simulink model "euler_dynamics"  (R2024b)
settings: Solver=FixedStepAuto  StartTime=0.0  StopTime=1500  FixedStep=0.1  RelTol=1e-6  AbsTol=1e-6
values from neighbouring files (symbols this model uses):
  com_0 = [0,0,0]    [Specefications.m]
  com_1 = [60,60,60]*deg    [Specefications.m]
  com_2 = [-60,-60,-60]*deg    [Specefications.m]
  com_3 = [0,0,0]*deg    [Specefications.m]
  deg = pi/180    (= 0.0174532925199)    [Specefications.m]
  initial_euler_angles = [30,30,30].*deg    [Specefications.m]
  J = diag([J11,J22,J33])    [Specefications.m]
  K_e = lqr(Linearized_model_e,Q,R)    [Linear_controller_design.m]
  n = (mu_Earth/r^3).^0.5    [Specefications.m]
  t_d = [1e-4,1e-4,1e-4]    [Specefications.m]
  w = [0,0,0].*deg    [Specefications.m]
libraries: matrix_library x2, sharedtransform x2
settings Model: Creator=diogo  LastModifiedBy=diogo

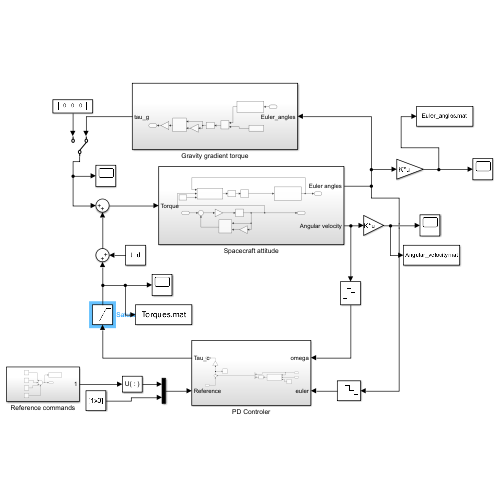
[thumbnail: Simulink's stored preview of the top-level diagram]
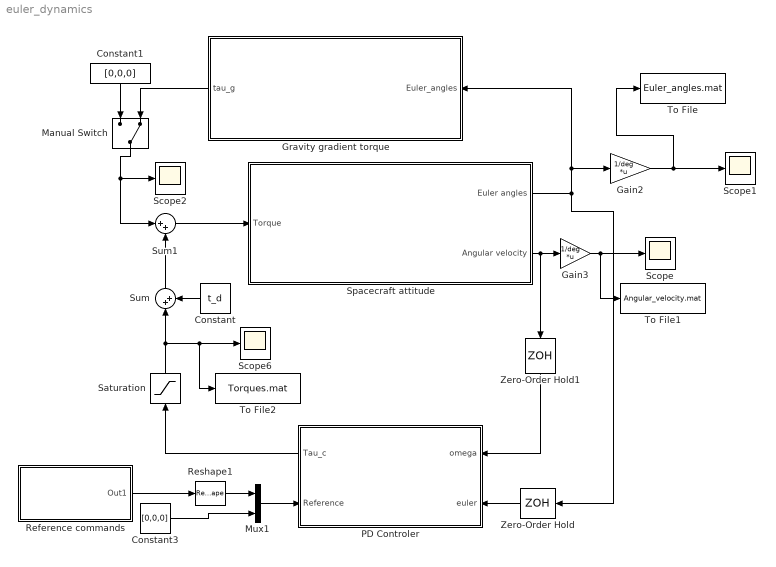
== system euler_dynamics ==
  Constant : Constant  Value=t_d
  Constant1 : Constant  Value=[0,0,0]
  Constant3 : Constant  Value=[0,0,0]
  Gain2 : Gain  Gain=1/deg  Multiplication=Matrix(K*u)
  Gain3 : Gain  Gain=1/deg  Multiplication=Matrix(K*u)
  Gravity gradient torque : Subsystem
  Manual Switch : ManualSwitch  CurrentSetting=0
  Mux1 : Mux  Inputs=2
  PD Controler : Subsystem
      settings: PortSchema="{\"entries\":[{\"content\":{\"sides\":[{\"content\":{\"connectorIds\":[\"Out1\",\"In1\"]},\"type\":\"ConnectorPlacement.EquallySpacedRectSide\",\"uuid\":\"f595316a-67fa-4e45-afef-328468ac5eb6\"},{\"content\":{\"connectorIds\":[\"In2\",\"In3\"],\"side\":\"RIGHT\"},\"type\":\"ConnectorPlacement.EquallySpacedRectSide\",\"uuid\":\"1d08d35b-debb-44a1-b4ca-ee5ff70ce730\"},{\"content\":{\"side\":\"TOP\"},\"type\":\"ConnectorPlacement.EquallySpacedRectSide\",\"uuid\":\"f0dda074-91f8-4f2d-97e8-f0eac84287d6\"}]},\"type\":\"ConnectorPlacement.EquallySpacedConnector\",\"uuid\":\"e9b94e59-1199-495c-ac6d-8aec278c5c81\"}],\"packageUris\":[\"http://schema.mathworks.com/mf0/Connector/R2020b\"],\"version\":\"1.0\"}"
  Reference commands : Subsystem
  Reshape1 : Reshape
  Saturation : Saturate  UpperLimit=1  LowerLimit=-1
  Scope{,1..2,6} (4 alike) : Scope
  Spacecraft attitude : Subsystem
  Sum : Sum  Inputs=|++
  Sum1 : Sum  Inputs=|++
  To File : ToFile  Filename=Euler_angles.mat  MatrixName=values  SaveFormat=Timeseries
  To File1 : ToFile  Filename=Angular_velocity.mat  MatrixName=values  SaveFormat=Timeseries
  To File2 : ToFile  Filename=Torques.mat  MatrixName=values  SaveFormat=Timeseries
  Zero-Order Hold : ZeroOrderHold  SampleTime=0.1
  Zero-Order Hold1 : ZeroOrderHold  SampleTime=0.1
  wires:
  Gain3/1 -> To File1/1, Scope/1
  Spacecraft attitude/2(Angular velocity) -> Zero-Order Hold1/1, Gain3/1
  Constant/1 -> Sum/2
  Sum/1 -> Sum1/2
  Sum1/1 -> Spacecraft attitude/1(Torque)
  Gain2/1 -> To File/1, Scope1/1
  Constant1/1 -> Manual Switch/1
  Gravity gradient torque/1(tau_g) -> Manual Switch/2
  Manual Switch/1 -> Sum1/1, Scope2/1
  Spacecraft attitude/1(Euler angles) -> Gain2/1, Gravity gradient torque/1(Euler_angles), Zero-Order Hold/1
  Reference commands/1(Out1) -> Reshape1/1
  Reshape1/1 -> Mux1/1
  Constant3/1 -> Mux1/2
  PD Controler/1(Tau_c) -> Saturation/1
  Zero-Order Hold1/1 -> PD Controler/2(omega)
  Zero-Order Hold/1 -> PD Controler/3(euler)
  Mux1/1 -> PD Controler/1(Reference)
  Saturation/1 -> Sum/1, To File2/1, Scope6/1

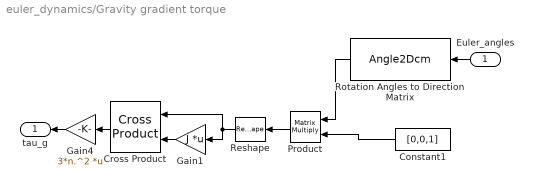
== system euler_dynamics/Gravity gradient torque ==
  Euler_angles : Inport
  Constant1 : Constant  Value=[0,0,1]
  Cross Product : matrix_library/Cross Product
  Gain1 : Gain  Gain=J  Multiplication=Matrix(K*u)
  Gain4 : Gain  Gain=3*n.^2  Multiplication=Matrix(K*u)
  Product : Product  Multiplication=Matrix(*)
  Reshape : Reshape
  Rotation Angles to Direction  Matrix : Angle2Dcm
      settings: AttributesFormatString=Rotation Order: %<rotationOrder>
  tau_g : Outport
  wires:
  Constant1/1 -> Product/2
  Gain1/1 -> Cross Product/2
  Gain4/1 -> tau_g/1
  Cross Product/1 -> Gain4/1
  Euler_angles/1 -> Rotation Angles to Direction  Matrix/1
  Product/1 -> Reshape/1
  Reshape/1 -> Gain1/1, Cross Product/1
  Rotation Angles to Direction  Matrix/1 -> Product/1

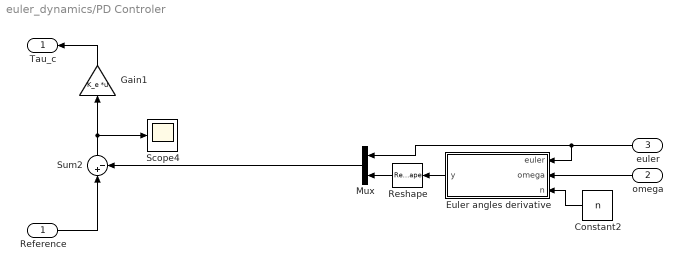
== system euler_dynamics/PD Controler ==
  Reference : Inport
  omega : Inport  Port=2
  euler : Inport  Port=3
  Constant2 : Constant  Value=n
  Euler angles derivative : MATLAB Function  TreatAsAtomicUnit=on
  Gain1 : Gain  Gain=K_e  Multiplication=Matrix(K*u)
  Mux : Mux  Inputs=2
  Reshape : Reshape
  Scope4 : Scope
  Sum2 : Sum  Inputs=|+-
  Tau_c : Outport
  wires:
  Sum2/1 -> Scope4/1, Gain1/1
  Constant2/1 -> Euler angles derivative/3(n)
  Mux/1 -> Sum2/2
  euler/1 -> Mux/1, Euler angles derivative/1(euler)
  Reshape/1 -> Mux/2
  Euler angles derivative/1(y) -> Reshape/1
  Gain1/1 -> Tau_c/1
  omega/1 -> Euler angles derivative/2(omega)
  Reference/1 -> Sum2/1

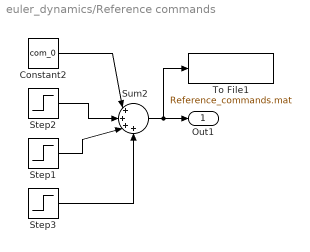
== system euler_dynamics/Reference commands ==
  Constant2 : Constant  Value=com_0
  Step1 : Step  Time=500.1  After=com_2 - com_1  SampleTime=0  VectorParams1D=off
  Step2 : Step  Time=100  After=com_1 - com_0  SampleTime=0  VectorParams1D=off
  Step3 : Step  Time=900.1  After=com_3 - com_2  SampleTime=0  VectorParams1D=off
  Sum2 : Sum  Inputs=|++++
  To File1 : ToFile  Filename=Reference_commands.mat  MatrixName=values  SaveFormat=Timeseries
  Out1 : Outport
  wires:
  Step3/1 -> Sum2/4
  Step1/1 -> Sum2/3
  Step2/1 -> Sum2/2
  Constant2/1 -> Sum2/1
  Sum2/1 -> To File1/1, Out1/1

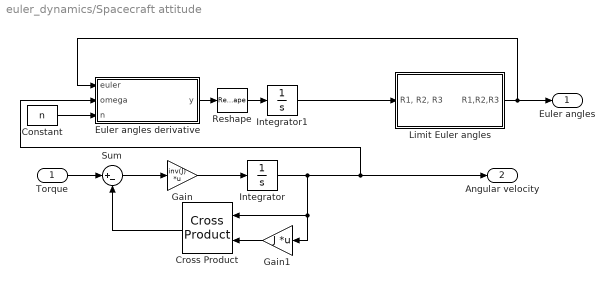
== system euler_dynamics/Spacecraft attitude ==
  Torque : Inport
  Constant : Constant  Value=n
  Cross Product : matrix_library/Cross Product
  Euler angles derivative : MATLAB Function  TreatAsAtomicUnit=on
  Gain : Gain  Gain=inv(J)  Multiplication=Matrix(K*u)
  Gain1 : Gain  Gain=J  Multiplication=Matrix(K*u)
  Integrator : Integrator  InitialCondition=w
  Integrator1 : Integrator  InitialCondition=initial_euler_angles
  Limit Euler angles : Subsystem
  Reshape : Reshape
  Sum : Sum  Inputs=|+-
  Euler angles : Outport
  Angular velocity : Outport  Port=2
  wires:
  Gain1/1 -> Cross Product/2
  Integrator/1 -> Cross Product/1, Gain1/1, Euler angles derivative/2(omega), Angular velocity/1
  Sum/1 -> Gain/1
  Cross Product/1 -> Sum/2
  Gain/1 -> Integrator/1
  Torque/1 -> Sum/1
  Euler angles derivative/1(y) -> Reshape/1
  Integrator1/1 -> Limit Euler angles/1("R1, R2, R3")
  Constant/1 -> Euler angles derivative/3(n)
  Limit Euler angles/1(R1,R2,R3) -> Euler angles derivative/1(euler), Euler angles/1
  Reshape/1 -> Integrator1/1

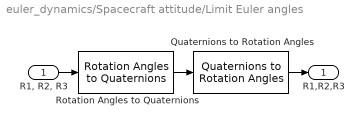
== system euler_dynamics/Spacecraft attitude/Limit Euler angles ==
  "R1, R2, R3" : Inport
  Quaternions to Rotation Angles : sharedtransform/Quaternions to Rotation Angles  rotationOrder=ZYX  aMode=aMode
  Rotation Angles to Quaternions : sharedtransform/Rotation Angles to Quaternions  rotationOrder=ZYX  aMode=aMode
  R1,R2,R3 : Outport
  wires:
  Quaternions to Rotation Angles/1 -> R1,R2,R3/1
  Rotation Angles to Quaternions/1 -> Quaternions to Rotation Angles/1
  "R1, R2, R3"/1 -> Rotation Angles to Quaternions/1

== matlab function euler_dynamics/Spacecraft attitude/Euler angles derivative ==
  data: euler input; y output; omega input; n input
function y = fcn(euler,omega,n)
theta = euler(2);
phi = euler(3);
psi = euler(1);
mat = (1/cos(theta))*[cos(theta),sin(phi)*sin(theta),cos(phi)*sin(theta);
0, cos(phi)*cos(theta),-sin(phi)*cos(theta);
0, sin(phi), cos(phi)
];
z = mat*omega + n/cos(theta)*[sin(psi); cos(theta)*cos(psi); sin(theta)*sin(psi)];
y = [z(3),z(2),z(1)];

== matlab function euler_dynamics/PD Controler/Euler angles derivative ==
  data: euler input; y output; omega input; n input
function y = fcn(euler,omega,n)
theta = euler(2);
phi = euler(3);
psi = euler(1);
mat = (1/cos(theta))*[cos(theta),sin(phi)*sin(theta),cos(phi)*sin(theta);
0, cos(phi)*cos(theta),-sin(phi)*cos(theta);
0, sin(phi), cos(phi)
];
z = mat*omega + n/cos(theta)*[sin(psi); cos(theta)*cos(psi); sin(theta)*sin(psi)];
y = [z(3),z(2),z(1)];
